simulink model "prob2"  (R2020b)
settings: Solver=VariableStepAuto  StartTime=0.0  StopTime=100  RelTol=1e-3
settings Model: Creator=DELL  LastModifiedBy=DELL

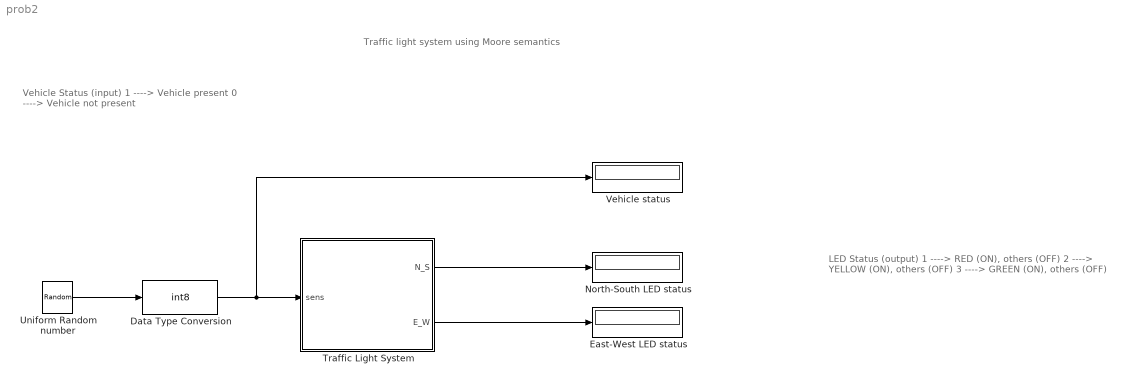
== system prob2 ==
  note: Traffic light system using Moore semantics
  note: Vehicle Status (input)
      |
      | 1 ----> Vehicle present
      | 0 ----> Vehicle not present
  note: LED Status (output)
      |
      | 1 ----> RED (ON), others (OFF)
      | 2 ----> YELLOW (ON), others (OFF)
      | 3 ----> GREEN (ON), others (OFF)
  Data Type Conversion : DataTypeConversion  OutDataTypeStr=int8  RndMeth=Nearest
  East-West LED status : Display
  North-South LED status : Display
  Traffic Light System : Stateflow chart  TreatAsAtomicUnit=on
  Uniform Random number : UniformRandomNumber  Minimum=0  SampleTime=0.25
  Vehicle status : Display
  wires:
  Traffic Light System/1(N_S) -> North-South LED status/1
  Traffic Light System/2(E_W) -> East-West LED status/1
  Uniform Random number/1 -> Data Type Conversion/1
  Data Type Conversion/1 -> Vehicle status/1, Traffic Light System/1(sens)

== stateflow chart prob2/Traffic Light System ==
  state Stop_to_Go
    N_S=RED;
    E_W=YELLOW;
  state Stop
    N_S=RED;
    E_W=GREEN;
  state Stop_for_Traffic
    N_S=RED;
    E_W=GREEN;
  state Go_to_Stop
    N_S=YELLOW;
    E_W=RED;
  state Go
    N_S=GREEN;
    E_W=RED;
  (default) -> Stop
  Stop -> Stop_for_Traffic : after(20,tick)
  Stop_for_Traffic -> Stop_to_Go : [sens]
  Go_to_Stop -> Stop : after(3,tick)
  Stop_to_Go -> Go : after(3,tick)
  Go -> Go_to_Stop : after(10,tick)
  data: sens input; N_S output; E_W output; GREEN constant double =3; RED constant double =1; YELLOW constant double =2
